simulink model "non_linear_model"  (R2021b)
settings: Solver=VariableStepAuto  StartTime=0.0  StopTime=10.0  RelTol=1e-3
settings Model: Creator=peterkrull  LastModifiedBy=peterkrull

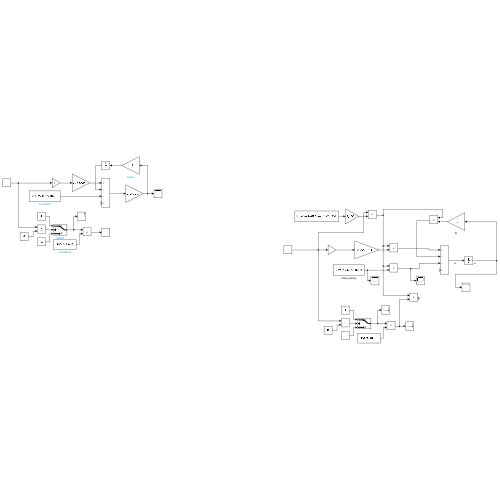
[thumbnail: Simulink's stored preview of the top-level diagram]
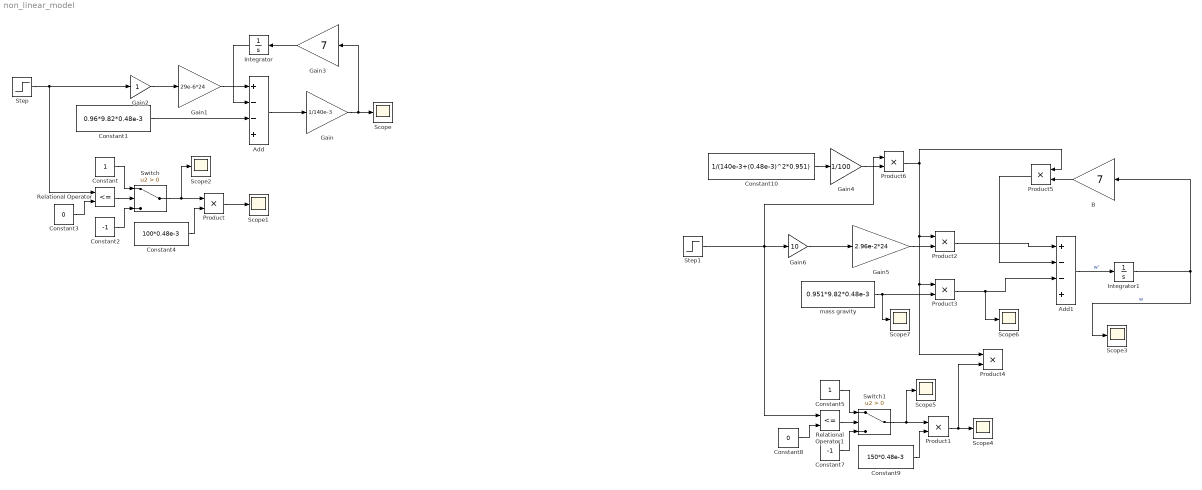
== system non_linear_model ==
  Add : Sum  Inputs=+--+
  Add1 : Sum  Inputs=+--+
  B : Gain  Gain=7
  Constant : Constant
  Constant1 : Constant  Value=0.96*9.82*0.48e-3
  Constant10 : Constant  Value=1/(140e-3+(0.48e-3)^2*0.951)
  Constant2 : Constant  Value=-1
  Constant3 : Constant  Value=0
  Constant4 : Constant  Value=100*0.48e-3
  Constant5 : Constant
  Constant7 : Constant  Value=-1
  Constant8 : Constant  Value=0
  Constant9 : Constant  Value=150*0.48e-3
  Gain : Gain  Gain=1/140e-3
  Gain1 : Gain  Gain=29e-6*24
  Gain2 : Gain
  Gain3 : Gain  Gain=7
  Gain4 : Gain  Gain=1/100
  Gain5 : Gain  Gain=2.96e-2*24
  Gain6 : Gain  Gain=10
  Integrator : Integrator
  Integrator1 : Integrator
  Product{,1..6} (7 alike) : Product
  Relational Operator : RelationalOperator  Operator=<=  OutDataTypeStr=boolean  RndMeth=Simplest
  Relational Operator1 : RelationalOperator  Operator=<=  OutDataTypeStr=boolean  RndMeth=Simplest
  Scope{,1..7} (8 alike) : Scope
  Step : Step  SampleTime=0
  Step1 : Step  Before=0.1  SampleTime=0
  Switch : Switch  Criteria=u2 > Threshold
  Switch1 : Switch  Criteria=u2 > Threshold
  mass gravity : Constant  Value=0.951*9.82*0.48e-3
  wires:
  Gain/1 -> Gain3/1, Scope/1
  Add/1 -> Gain/1
  Gain1/1 -> Add/1
  Step/1 -> Relational Operator/1, Gain2/1
  Gain2/1 -> Gain1/1
  Integrator/1 -> Add/2
  Constant1/1 -> Add/3
  Relational Operator/1 -> Switch/2
  Constant2/1 -> Switch/3
  Constant/1 -> Switch/1
  Constant3/1 -> Relational Operator/2
  Switch/1 -> Scope2/1, Product/1
  Constant4/1 -> Product/2
  Gain3/1 -> Integrator/1
  Product/1 -> Scope1/1
  Constant8/1 -> Relational Operator1/2
  Constant9/1 -> Product1/2
  Step1/1 -> Relational Operator1/1, Product6/1, Gain6/1
  Constant5/1 -> Switch1/1
  Product1/1 -> Product4/2, Scope4/1
  Constant7/1 -> Switch1/3
  Switch1/1 -> Scope5/1, Product1/1
  Relational Operator1/1 -> Switch1/2
  Integrator1/1 -> Scope3/1, B/1  "w"
  Add1/1 -> Integrator1/1  "w'"
  Gain5/1 -> Product2/2
  mass gravity/1 -> Scope7/1, Product3/2
  Product5/1 -> Add1/2
  Constant10/1 -> Gain4/1
  B/1 -> Product5/2
  Product6/1 -> Product5/1, Product4/1, Product3/1, Product2/1
  Product3/1 -> Scope6/1, Add1/3
  Gain4/1 -> Product6/2
  Gain6/1 -> Gain5/1
  Product2/1 -> Add1/1
